simulink library "INT_CnvLead_Trq2Q"  (R2016b)
settings: Solver=VariableStepAuto  StartTime=0.0  StopTime=10.0  RelTol=1e-3
settings Model: Creator=zhoutinglin  LastModifiedBy=zhoutinglin

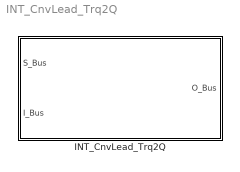
== system INT_CnvLead_Trq2Q ==
  INT_CnvLead_Trq2Q : Subsystem

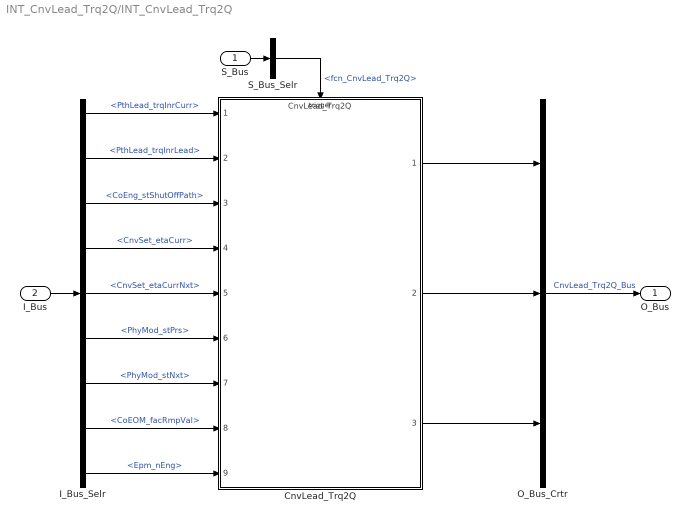
== system INT_CnvLead_Trq2Q/INT_CnvLead_Trq2Q ==
  S_Bus : Inport
  I_Bus : Inport  Port=2
  CnvLead_Trq2Q : ModelReference  ModelNameDialog=CnvLead_Trq2Q  SimulationMode=Normal  ModelReferenceVersion=1.37  TriggerPortName=function  TriggerPortTriggerType=function-call  TriggerPortStatesWhenEnabling=held
  I_Bus_Selr : BusSelector  OutputSignals=PthLead_trqInrCurr,PthLead_trqInrLead,CoEng_stShutOffPath,CnvSet_etaCurr,CnvSet_etaCurrNxt,PhyMod_stPrs,PhyMod_stNxt,CoEOM_facRmpVal,Epm_nEng
  O_Bus_Crtr : BusCreator  Inputs=3
  S_Bus_Selr : BusSelector  OutputSignals=fcn_CnvLead_Trq2Q
  O_Bus : Outport
  wires:
  S_Bus_Selr/1 -> CnvLead_Trq2Q/Trigger  "<fcn_CnvLead_Trq2Q>"
  S_Bus/1 -> S_Bus_Selr/1
  I_Bus/1 -> I_Bus_Selr/1
  I_Bus_Selr/1 -> CnvLead_Trq2Q/1  "<PthLead_trqInrCurr>"
  I_Bus_Selr/2 -> CnvLead_Trq2Q/2  "<PthLead_trqInrLead>"
  I_Bus_Selr/3 -> CnvLead_Trq2Q/3  "<CoEng_stShutOffPath>"
  I_Bus_Selr/4 -> CnvLead_Trq2Q/4  "<CnvSet_etaCurr>"
  I_Bus_Selr/5 -> CnvLead_Trq2Q/5  "<CnvSet_etaCurrNxt>"
  I_Bus_Selr/6 -> CnvLead_Trq2Q/6  "<PhyMod_stPrs>"
  I_Bus_Selr/7 -> CnvLead_Trq2Q/7  "<PhyMod_stNxt>"
  I_Bus_Selr/8 -> CnvLead_Trq2Q/8  "<CoEOM_facRmpVal>"
  I_Bus_Selr/9 -> CnvLead_Trq2Q/9  "<Epm_nEng>"
  O_Bus_Crtr/1 -> O_Bus/1  "CnvLead_Trq2Q_Bus"
  CnvLead_Trq2Q/1 -> O_Bus_Crtr/1
  CnvLead_Trq2Q/2 -> O_Bus_Crtr/2
  CnvLead_Trq2Q/3 -> O_Bus_Crtr/3
